simulink model "Task5"  (R2019b)
settings: Solver=VariableStepAuto  StartTime=0.0  StopTime=10.0  RelTol=1e-3
libraries: simulink x2
settings Model: Creator=12393  LastModifiedBy=12393

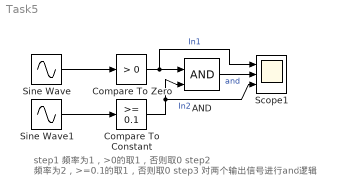
== system Task5 ==
  note: step1 频率为1，>0的取1，否则取0
      | step2 频率为2，>=0.1的取1，否则取0
      | step3 对两个输出信号进行and逻辑
  AND : Logic  IconShape=distinctive  AllPortsSameDT=off  OutDataTypeStr=boolean
  Compare To Constant : simulink/Logic and Bit Operations/Compare To Constant  relop=>=  const=0.1  OutDataTypeStr=boolean
  Compare To Zero : simulink/Logic and Bit Operations/Compare To Zero  relop=>  OutDataTypeStr=boolean
  Scope1 : Scope  NumInputPorts=3
  Sine Wave : Sin  SampleTime=0
      settings: AttributesFormatString=Frequency=%<Frequency> rad/sec
  Sine Wave1 : Sin  Frequency=2  SampleTime=0
      settings: AttributesFormatString=Frequency=%<Frequency> rad/sec
  wires:
  Sine Wave1/1 -> Compare To Constant/1
  AND/1 -> Scope1/2  "and"
  Compare To Constant/1 -> Scope1/3, AND/2  "In2"
  Compare To Zero/1 -> Scope1/1, AND/1  "In1"
  Sine Wave/1 -> Compare To Zero/1
